simulink model "CS_PVr"  (R2014b)
settings: Solver=FixedStepDiscrete  StartTime=0.0  StopTime=Te  FixedStep=Tm  RelTol=1e-3
StopFcn:
  | salida(simout)
undefined symbols (not defined in the file): A, B, Dp, Dv, Fcdp, Fcdv, Fcp, Fcv, Humusoft, Ip, Iv, Kbp, Kbv, MF624, Np, Nv, Pf, Pi, Pp, Pv, Tm, Tp
libraries: rtwinlib x3
settings Model: SimulationMode=external  ExtModeTrigDuration=100000  Creator=Equipo-Servo  LastModifiedBy=Servo
settings DebuggingCC: UnderspecifiedInitializationDetection=Classic  MergeDetectMultiDrivingBlocksExec=none  StateNameClashWarn=warning
settings HardwareCC: ProdIntDivRoundTo=Zero  ProdEndianess=LittleEndian  ProdHWDeviceType=Generic->32-bit x86 compatible
settings RTWCC: SystemTargetFile=rtwin.tlc  TemplateMakefile=rtwin.tmf  Description=Real-Time Windows Target  ProcessScript=rtwin_make_rtw_hook  RTWCompilerOptimization=On
settings CodeAppCC: MaxIdLength=95
settings RTWinTargetCC: TargetLibSuffix=_rtwin.lib  TargetPreCompLibLocation=C:\Program Files\MATLAB\R2014b\toolbox\rtw\targets\rtwin\lib\win64

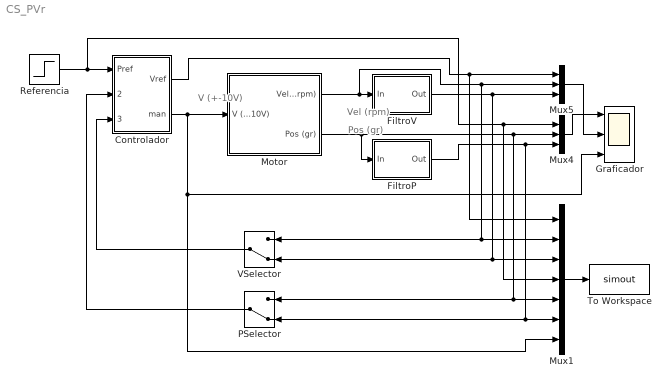
== system CS_PVr ==
  note: Vel
      | (rpm)
  note: Pos
      | (gr)
  note: V (+-10V)
  Controlador : Subsystem  mask{T=Tm, Pp=Pp, Ip=Ip, Kbp=Kbp, Dp=Dp, Fcdp=Fcdp, Pv=Pv, Iv=Iv, Kbv=Kbv, Dv=Dv, Fcdv=Fcdv}
      mask prompts: T "Período de muestreo"; Kbp "Kbp (anti windup)"; Fcdp "Fcdp (Hz)"; Kbv "Kbv (anti windup)"; Fcdv "Fcdv (Hz)"
      mask init:
      | Np = 2*pi*Fcdp;
      | Nv = 2*pi*Fcdv;
  FiltroP : Subsystem  mask{N=Np, Fc=Fcp, Fm=1/Tm}
      mask prompts: N "Orden del filtro (Butterworth)"; Fc "Frecuencia de corte (Fc<Fm/2)"; Fm "Frecuencia de muestreo"
      mask init:
      | Fn = Fm/2;   % Frecuencia de Nyquist
      | [B,A] = butter(N,Fc/Fn);
  FiltroV : Subsystem  mask{N=Nv, Fc=Fcv, Fm=1/Tm}
      mask prompts: N "Orden del filtro (Butterworth)"; Fc "Frecuencia de corte (Fc<Fm/2)"; Fm "Frecuencia de muestreo"
      mask init:
      | Fn = Fm/2;   % Frecuencia de Nyquist
      | [B,A] = butter(N,Fc/Fn);
  Graficador : Scope  NumInputPorts=3
      settings: TimeRange=10  YMin=-100~-100~-30  YMax=100~100~30  SampleTime=Tm
  Motor : Subsystem
  Mux1 : Mux  Inputs=7
  Mux4 : Mux  Inputs=3
  Mux5 : Mux  Inputs=3
  PSelector : ManualSwitch  CurrentSetting=0
  Referencia : Step  Time=Tp  Before=Pi  After=Pf  SampleTime=0
  To Workspace : ToWorkspace  VariableName=simout  SaveFormat=Structure With Time  SampleTime=Tm
  VSelector : ManualSwitch  CurrentSetting=0
  wires:
  Motor/2(Pos (gr)) -> FiltroP/1(In), Mux4/2, PSelector/1, Mux1/5
  Referencia/1 -> Controlador/1(Pref), Mux1/4, Mux4/1
  FiltroP/1(Out) -> Mux4/3, PSelector/2, Mux1/6
  PSelector/1 -> Controlador/2(Pmed)
  Controlador/2(man) -> Mux1/7, Graficador/3, Motor/1(V (+-10V))
  Motor/1(Vel (rpm)) -> Mux1/2, VSelector/1, Mux5/2, FiltroV/1(In)
  FiltroV/1(Out) -> VSelector/2, Mux1/3, Mux5/3
  Controlador/1(Vref) -> Mux1/1, Mux5/1
  VSelector/1 -> Controlador/3(Vmed)
  Mux1/1 -> To Workspace/1
  Mux4/1 -> Graficador/1
  Mux5/1 -> Graficador/2

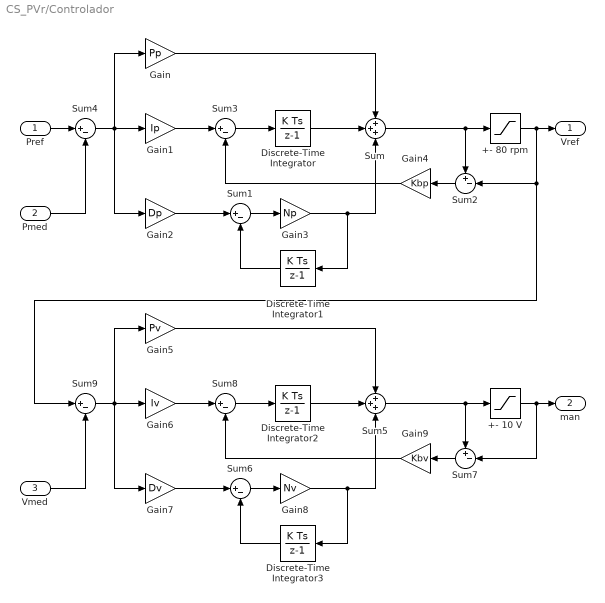
== system CS_PVr/Controlador ==
  Pref : Inport
  Pmed : Inport  Port=2
  Vmed : Inport  Port=3
  +- 10 V : Saturate  UpperLimit=10  LowerLimit=-10
  +- 80 rpm : Saturate  UpperLimit=80  LowerLimit=-80
  Discrete-Time Integrator{,1..3} (4 alike) : DiscreteIntegrator  SampleTime=T
  Gain : Gain  Gain=Pp
  Gain1 : Gain  Gain=Ip
  Gain2 : Gain  Gain=Dp
  Gain3 : Gain  Gain=Np
  Gain4 : Gain  Gain=Kbp
  Gain5 : Gain  Gain=Pv
  Gain6 : Gain  Gain=Iv
  Gain7 : Gain  Gain=Dv
  Gain8 : Gain  Gain=Nv
  Gain9 : Gain  Gain=Kbv
  Sum : Sum  Inputs=+++
  Sum{1,3..4,6,8..9} (6 alike) : Sum  Inputs=|+-
  Sum2 : Sum  Inputs=+-|
  Sum5 : Sum  Inputs=+++
  Sum7 : Sum  Inputs=+-|
  Vref : Outport
  man : Outport  Port=2
  wires:
  Sum/1 -> Sum2/1, +- 80 rpm/1
  Gain/1 -> Sum/1
  Discrete-Time Integrator/1 -> Sum/2
  Pref/1 -> Sum4/1
  Sum1/1 -> Gain3/1
  Gain2/1 -> Sum1/1
  Discrete-Time Integrator1/1 -> Sum1/2
  Gain3/1 -> Sum/3, Discrete-Time Integrator1/1
  Sum2/1 -> Gain4/1
  Sum3/1 -> Discrete-Time Integrator/1
  Gain1/1 -> Sum3/1
  Gain4/1 -> Sum3/2
  Sum4/1 -> Gain2/1, Gain/1, Gain1/1
  Pmed/1 -> Sum4/2
  Sum5/1 -> +- 10 V/1, Sum7/1
  +- 10 V/1 -> man/1, Sum7/2
  Gain5/1 -> Sum5/1
  Discrete-Time Integrator2/1 -> Sum5/2
  +- 80 rpm/1 -> Sum9/1, Sum2/2, Vref/1
  Sum6/1 -> Gain8/1
  Gain7/1 -> Sum6/1
  Discrete-Time Integrator3/1 -> Sum6/2
  Gain8/1 -> Discrete-Time Integrator3/1, Sum5/3
  Sum7/1 -> Gain9/1
  Sum8/1 -> Discrete-Time Integrator2/1
  Gain6/1 -> Sum8/1
  Gain9/1 -> Sum8/2
  Sum9/1 -> Gain7/1, Gain6/1, Gain5/1
  Vmed/1 -> Sum9/2

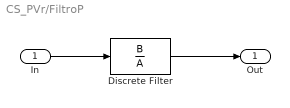
== system CS_PVr/FiltroP ==
  In : Inport
  Discrete Filter : DiscreteFilter  Numerator=B  Denominator=A  SampleTime=1/Fm
  Out : Outport
  wires:
  Discrete Filter/1 -> Out/1
  In/1 -> Discrete Filter/1

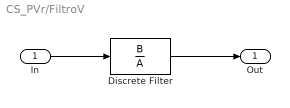
== system CS_PVr/FiltroV ==
  In : Inport
  Discrete Filter : DiscreteFilter  Numerator=B  Denominator=A  SampleTime=1/Fm
  Out : Outport
  wires:
  In/1 -> Discrete Filter/1
  Discrete Filter/1 -> Out/1

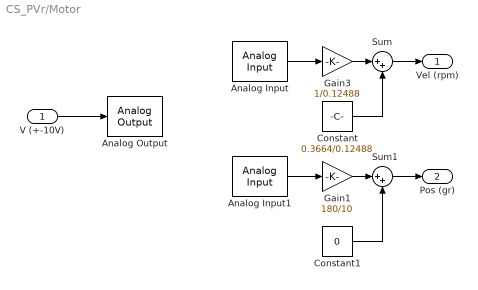
== system CS_PVr/Motor ==
  V (+-10V) : Inport
  Analog Input : rtwinlib/Analog Input  SampleTime=Tm  MaxMissedTicks=10  ShowMissedTicks=off  YieldWhenWaiting=off  DrvName=Humusoft/MF624  DrvAddress=0  DrvOptions=0  Channels=1  RangeMode=1  VoltRange=1  DataType=1
      settings: AttributesFormatString=Humusoft\nMF624 [0h]
  Analog Input1 : rtwinlib/Analog Input  SampleTime=Tm  MaxMissedTicks=10  ShowMissedTicks=off  YieldWhenWaiting=off  DrvName=Humusoft/MF624  DrvAddress=0  DrvOptions=0  Channels=2  RangeMode=1  VoltRange=1  DataType=1
      settings: AttributesFormatString=Humusoft\nMF624 [0h]
  Analog Output : rtwinlib/Analog Output  SampleTime=Tm  MaxMissedTicks=10  ShowMissedTicks=off  YieldWhenWaiting=off  DrvName=Humusoft/MF624  DrvAddress=0  DrvOptions=0  Channels=1  RangeMode=1  VoltRange=1  InitialValue=0  FinalValue=0
      settings: AttributesFormatString=Humusoft\nMF624 [0h]
  Constant : Constant  Value=0.3664/0.12488
  Constant1 : Constant  Value=0
  Gain1 : Gain  Gain=180/10
  Gain3 : Gain  Gain=1/0.12488
  Sum : Sum  Inputs=|++
  Sum1 : Sum  Inputs=|++
  Vel (rpm) : Outport
  Pos (gr) : Outport  Port=2
  wires:
  V (+-10V)/1 -> Analog Output/1
  Analog Input/1 -> Gain3/1
  Constant/1 -> Sum/2
  Sum/1 -> Vel (rpm)/1
  Gain3/1 -> Sum/1
  Analog Input1/1 -> Gain1/1
  Constant1/1 -> Sum1/2
  Gain1/1 -> Sum1/1
  Sum1/1 -> Pos (gr)/1
